simulink subsystem "fuelTank"  (R2020b)
settings: Solver=VariableStepAuto  StartTime=0.0  StopTime=10.0  RelTol=1e-3
undefined symbols (not defined in the file): fuelCapacity
settings Model: Creator=mordi  LastModifiedBy=mordi

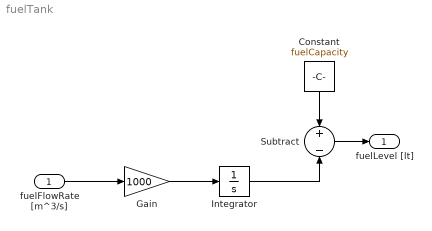
== system fuelTank ==
  fuelFlowRate [m^3/s] : Inport
  Constant : Constant  Value=fuelCapacity
  Gain : Gain  Gain=1000
  Integrator : Integrator
  Subtract : Sum  Inputs=+-
  fuelLevel [lt] : Outport
  wires:
  Constant/1 -> Subtract/1
  Integrator/1 -> Subtract/2
  Subtract/1 -> fuelLevel [lt]/1
  fuelFlowRate [m^3/s]/1 -> Gain/1
  Gain/1 -> Integrator/1
